simulink model "Final_10_26_SimulationProject"  (R2021a)
settings: Solver=VariableStepAuto  StartTime=0.0  StopTime=20  RelTol=1e-3
values from neighbouring files (symbols this model uses):
  A = [0,1,0,0 ... (first row only)    [Final_10_26_SimulationProject_Script.m]
  B = [0,0,0,0 ... (first row only)    [Final_10_26_SimulationProject_Script.m]
  C = [0 0 1 0 ... (first row only)    [Final_10_26_SimulationProject_Script.m]
  D = [0,0,0,0;0,0,0,0]    [Final_10_26_SimulationProject_Script.m]
settings Model: Creator=FOSTERPI  LastModifiedBy=FOSTERPI

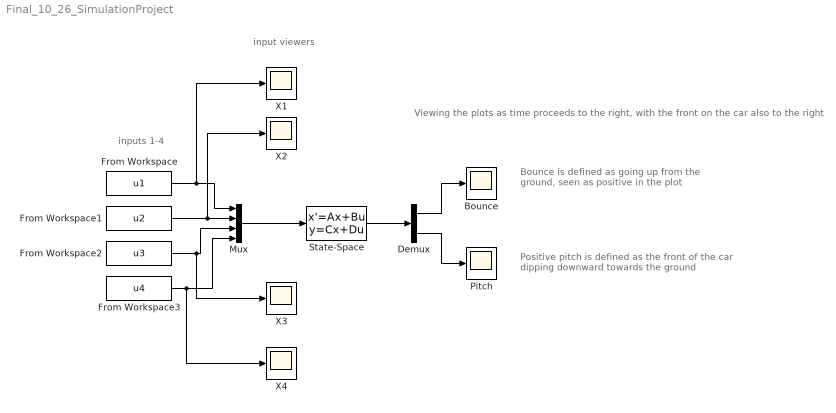
== system Final_10_26_SimulationProject ==
  note: Viewing the plots as time proceeds to the right, with the front on the car also to the right
  note: Bounce is defined as going up from the ground, seen as positive in the plot
  note: Positive pitch is defined as the front of the car dipping downward towards the ground
  note: input viewers
  note: inputs 1-4
  Bounce : Scope
  Demux : Demux  Outputs=2
  From Workspace : FromWorkspace  VariableName=u1  SampleTime=0.01
  From Workspace1 : FromWorkspace  VariableName=u2  SampleTime=0.01
  From Workspace2 : FromWorkspace  VariableName=u3  SampleTime=0.01
  From Workspace3 : FromWorkspace  VariableName=u4  SampleTime=0.01
  Mux : Mux
  Pitch : Scope
  State-Space : StateSpace  A=A  B=B  C=C  D=D  InitialCondition=0
  X{1..4} (4 alike) : Scope
  wires:
  State-Space/1 -> Demux/1
  Demux/1 -> Bounce/1
  Demux/2 -> Pitch/1
  Mux/1 -> State-Space/1
  From Workspace3/1 -> X4/1, Mux/4
  From Workspace/1 -> X1/1, Mux/1
  From Workspace2/1 -> X3/1, Mux/3
  From Workspace1/1 -> X2/1, Mux/2
